simulink library "andre_library"  (R2019b)
settings: Solver=VariableStepAuto  StartTime=0.0  StopTime=10.0  RelTol=1e-3
libraries: hdlsllib x3
settings Model: Creator=Yinglongli  LastModifiedBy=Yinglongli

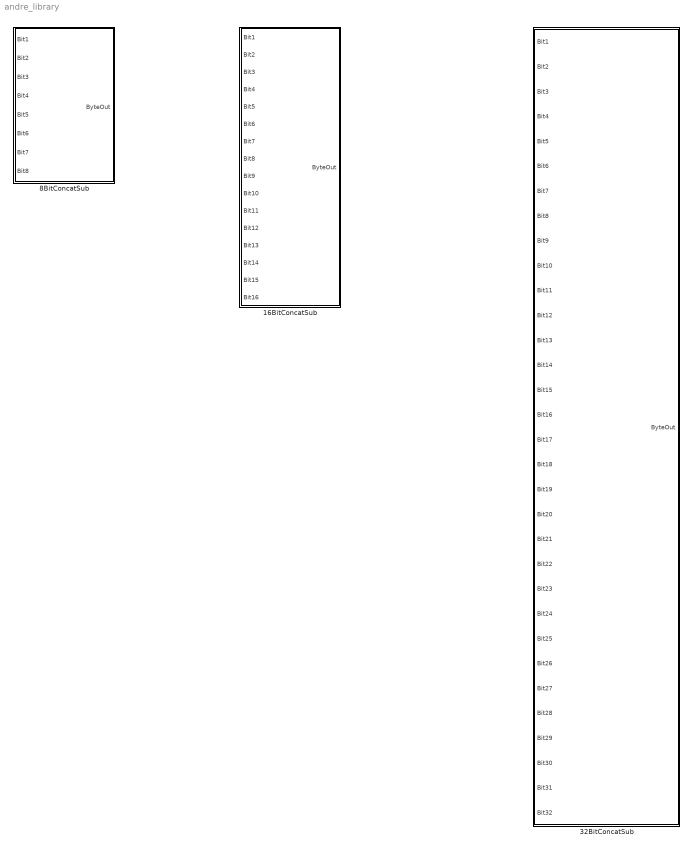
== system andre_library ==
  16BitConcatSub : Subsystem
  32BitConcatSub : Subsystem
  8BitConcatSub : Subsystem

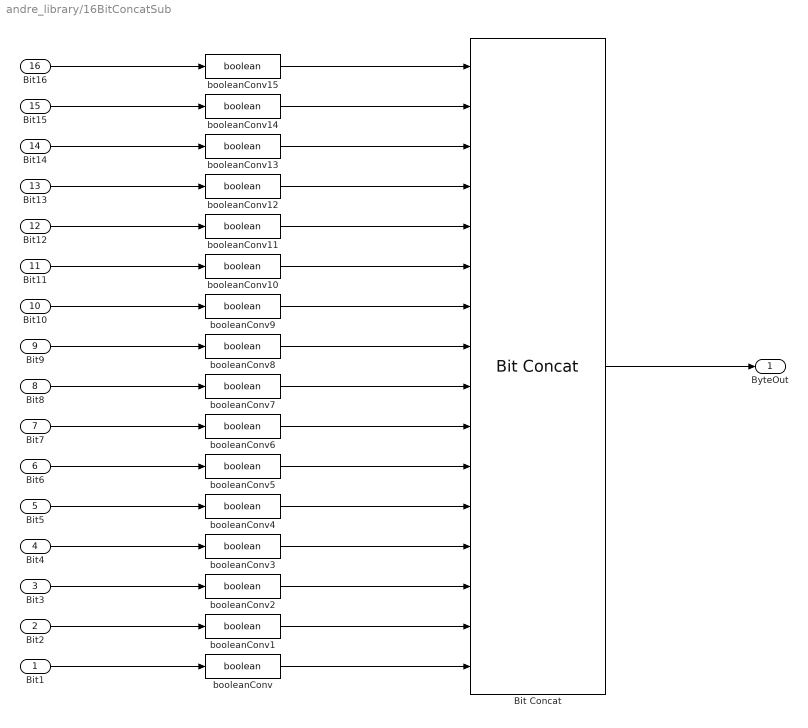
== system andre_library/16BitConcatSub ==
  Bit1 : Inport
  Bit2 : Inport  Port=2
  Bit3 : Inport  Port=3
  Bit4 : Inport  Port=4
  Bit5 : Inport  Port=5
  Bit6 : Inport  Port=6
  Bit7 : Inport  Port=7
  Bit8 : Inport  Port=8
  Bit9 : Inport  Port=9
  Bit10 : Inport  Port=10
  Bit11 : Inport  Port=11
  Bit12 : Inport  Port=12
  Bit13 : Inport  Port=13
  Bit14 : Inport  Port=14
  Bit15 : Inport  Port=15
  Bit16 : Inport  Port=16
  Bit Concat : hdlsllib/Logic and Bit Operations/Bit Concat  numInputs=16
      settings: SourceProductName=Simulink
  booleanConv{,1..15} (16 alike) : DataTypeConversion  OutDataTypeStr=boolean
  ByteOut : Outport
  wires:
  Bit Concat/1 -> ByteOut/1
  Bit8/1 -> booleanConv7/1
  Bit7/1 -> booleanConv6/1
  Bit6/1 -> booleanConv5/1
  Bit5/1 -> booleanConv4/1
  Bit4/1 -> booleanConv3/1
  Bit3/1 -> booleanConv2/1
  Bit2/1 -> booleanConv1/1
  Bit1/1 -> booleanConv/1
  booleanConv7/1 -> Bit Concat/9
  booleanConv6/1 -> Bit Concat/10
  booleanConv5/1 -> Bit Concat/11
  booleanConv4/1 -> Bit Concat/12
  booleanConv3/1 -> Bit Concat/13
  booleanConv2/1 -> Bit Concat/14
  booleanConv1/1 -> Bit Concat/15
  booleanConv/1 -> Bit Concat/16
  booleanConv15/1 -> Bit Concat/1
  booleanConv14/1 -> Bit Concat/2
  booleanConv13/1 -> Bit Concat/3
  booleanConv12/1 -> Bit Concat/4
  booleanConv11/1 -> Bit Concat/5
  booleanConv10/1 -> Bit Concat/6
  booleanConv9/1 -> Bit Concat/7
  booleanConv8/1 -> Bit Concat/8
  Bit16/1 -> booleanConv15/1
  Bit15/1 -> booleanConv14/1
  Bit14/1 -> booleanConv13/1
  Bit13/1 -> booleanConv12/1
  Bit12/1 -> booleanConv11/1
  Bit10/1 -> booleanConv9/1
  Bit11/1 -> booleanConv10/1
  Bit9/1 -> booleanConv8/1

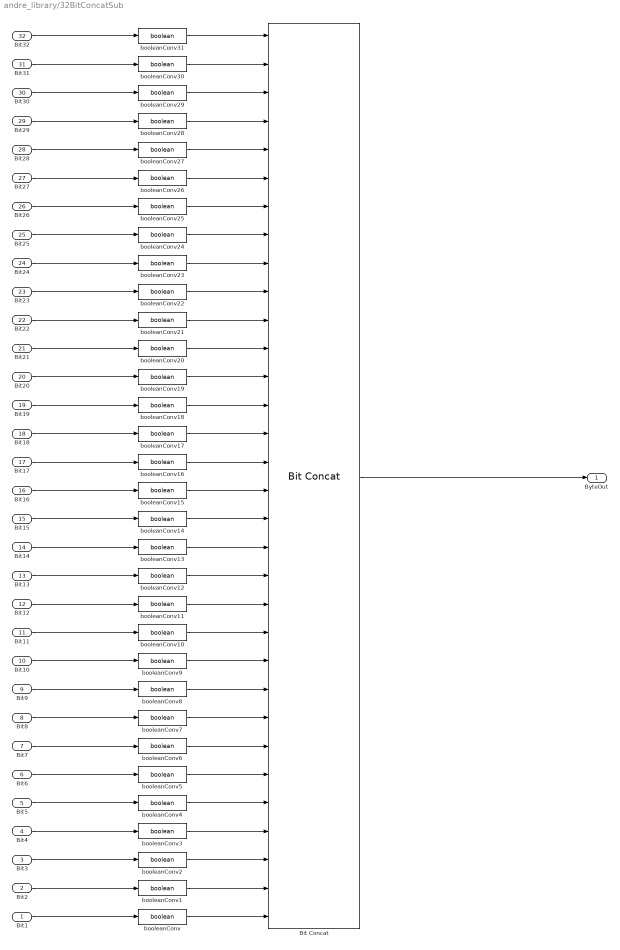
== system andre_library/32BitConcatSub ==
  Bit1 : Inport
  Bit2 : Inport  Port=2
  Bit3 : Inport  Port=3
  Bit4 : Inport  Port=4
  Bit5 : Inport  Port=5
  Bit6 : Inport  Port=6
  Bit7 : Inport  Port=7
  Bit8 : Inport  Port=8
  Bit9 : Inport  Port=9
  Bit10 : Inport  Port=10
  Bit11 : Inport  Port=11
  Bit12 : Inport  Port=12
  Bit13 : Inport  Port=13
  Bit14 : Inport  Port=14
  Bit15 : Inport  Port=15
  Bit16 : Inport  Port=16
  Bit17 : Inport  Port=17
  Bit18 : Inport  Port=18
  Bit19 : Inport  Port=19
  Bit20 : Inport  Port=20
  Bit21 : Inport  Port=21
  Bit22 : Inport  Port=22
  Bit23 : Inport  Port=23
  Bit24 : Inport  Port=24
  Bit25 : Inport  Port=25
  Bit26 : Inport  Port=26
  Bit27 : Inport  Port=27
  Bit28 : Inport  Port=28
  Bit29 : Inport  Port=29
  Bit30 : Inport  Port=30
  Bit31 : Inport  Port=31
  Bit32 : Inport  Port=32
  Bit Concat : hdlsllib/Logic and Bit Operations/Bit Concat  numInputs=32
      settings: SourceProductName=Simulink
  booleanConv{,1..31} (32 alike) : DataTypeConversion  OutDataTypeStr=boolean
  ByteOut : Outport
  wires:
  Bit Concat/1 -> ByteOut/1
  Bit8/1 -> booleanConv7/1
  Bit7/1 -> booleanConv6/1
  Bit6/1 -> booleanConv5/1
  Bit5/1 -> booleanConv4/1
  Bit4/1 -> booleanConv3/1
  Bit3/1 -> booleanConv2/1
  Bit2/1 -> booleanConv1/1
  Bit1/1 -> booleanConv/1
  Bit16/1 -> booleanConv15/1
  Bit15/1 -> booleanConv14/1
  Bit14/1 -> booleanConv13/1
  Bit13/1 -> booleanConv12/1
  Bit12/1 -> booleanConv11/1
  Bit10/1 -> booleanConv9/1
  Bit11/1 -> booleanConv10/1
  Bit9/1 -> booleanConv8/1
  booleanConv/1 -> Bit Concat/32
  booleanConv1/1 -> Bit Concat/31
  booleanConv2/1 -> Bit Concat/30
  booleanConv3/1 -> Bit Concat/29
  booleanConv4/1 -> Bit Concat/28
  booleanConv5/1 -> Bit Concat/27
  booleanConv6/1 -> Bit Concat/26
  booleanConv7/1 -> Bit Concat/25
  booleanConv8/1 -> Bit Concat/24
  booleanConv9/1 -> Bit Concat/23
  booleanConv10/1 -> Bit Concat/22
  booleanConv11/1 -> Bit Concat/21
  booleanConv12/1 -> Bit Concat/20
  booleanConv13/1 -> Bit Concat/19
  booleanConv14/1 -> Bit Concat/18
  booleanConv15/1 -> Bit Concat/17
  booleanConv31/1 -> Bit Concat/1
  booleanConv30/1 -> Bit Concat/2
  booleanConv29/1 -> Bit Concat/3
  booleanConv28/1 -> Bit Concat/4
  booleanConv27/1 -> Bit Concat/5
  booleanConv26/1 -> Bit Concat/6
  booleanConv25/1 -> Bit Concat/7
  booleanConv24/1 -> Bit Concat/8
  booleanConv23/1 -> Bit Concat/9
  booleanConv22/1 -> Bit Concat/10
  booleanConv21/1 -> Bit Concat/11
  booleanConv20/1 -> Bit Concat/12
  booleanConv19/1 -> Bit Concat/13
  booleanConv18/1 -> Bit Concat/14
  booleanConv17/1 -> Bit Concat/15
  booleanConv16/1 -> Bit Concat/16
  Bit17/1 -> booleanConv16/1
  Bit18/1 -> booleanConv17/1
  Bit19/1 -> booleanConv18/1
  Bit20/1 -> booleanConv19/1
  Bit21/1 -> booleanConv20/1
  Bit22/1 -> booleanConv21/1
  Bit23/1 -> booleanConv22/1
  Bit24/1 -> booleanConv23/1
  Bit25/1 -> booleanConv24/1
  Bit26/1 -> booleanConv25/1
  Bit27/1 -> booleanConv26/1
  Bit28/1 -> booleanConv27/1
  Bit29/1 -> booleanConv28/1
  Bit30/1 -> booleanConv29/1
  Bit31/1 -> booleanConv30/1
  Bit32/1 -> booleanConv31/1

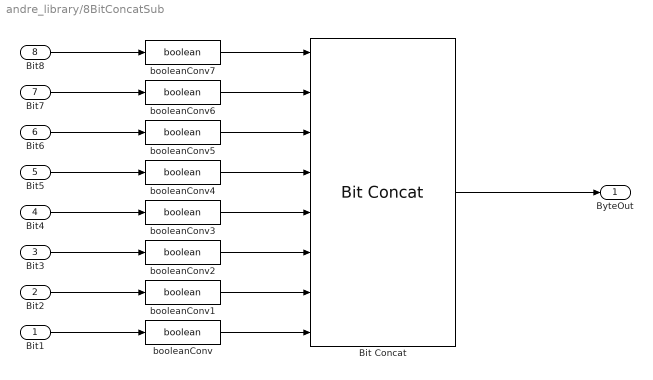
== system andre_library/8BitConcatSub ==
  Bit1 : Inport
  Bit2 : Inport  Port=2
  Bit3 : Inport  Port=3
  Bit4 : Inport  Port=4
  Bit5 : Inport  Port=5
  Bit6 : Inport  Port=6
  Bit7 : Inport  Port=7
  Bit8 : Inport  Port=8
  Bit Concat : hdlsllib/Logic and Bit Operations/Bit Concat  numInputs=8
      settings: SourceProductName=Simulink
  booleanConv{,1..7} (8 alike) : DataTypeConversion  OutDataTypeStr=boolean
  ByteOut : Outport
  wires:
  Bit Concat/1 -> ByteOut/1
  Bit8/1 -> booleanConv7/1
  Bit7/1 -> booleanConv6/1
  Bit6/1 -> booleanConv5/1
  Bit5/1 -> booleanConv4/1
  Bit4/1 -> booleanConv3/1
  Bit3/1 -> booleanConv2/1
  Bit2/1 -> booleanConv1/1
  Bit1/1 -> booleanConv/1
  booleanConv/1 -> Bit Concat/8
  booleanConv1/1 -> Bit Concat/7
  booleanConv2/1 -> Bit Concat/6
  booleanConv3/1 -> Bit Concat/5
  booleanConv4/1 -> Bit Concat/4
  booleanConv5/1 -> Bit Concat/3
  booleanConv6/1 -> Bit Concat/2
  booleanConv7/1 -> Bit Concat/1
